simulink model "pipeline_test25"  (Simulink 8.9)
settings: Solver=VariableStepAuto  StartTime=0.0  StopTime=190  RelTol=1e-3
libraries: xbsIndex_r4 x105
settings Model: Creator=jeenx  LastModifiedBy=jeenx
settings DataIOCC: LimitDataPoints=off  SaveFormat=Dataset  SignalLoggingSaveFormat=Dataset  ReturnWorkspaceOutputs=on
settings OptimizationCC: LifeSpan=auto
settings DebuggingCC: UnderspecifiedInitializationDetection=Simplified  MergeDetectMultiDrivingBlocksExec=error  FcnCallInpInsideContextMsg=error  StateNameClashWarn=none  SFUnexpectedBacktrackingDiag=error  SFNoUnconditionalDefaultTransitionDiag=error  SFExecutionAtInitializationDiag=warning
settings HardwareCC: ProdBitPerPointer=64  ProdBitPerSizeT=64  ProdBitPerPtrDiffT=64  ProdLargestAtomicFloat=Float  ProdIntDivRoundTo=Zero  ProdEndianess=LittleEndian  ProdWordSize=64  ProdHWDeviceType=Intel->x86-64 (Windows64)
settings ModelReferenceCC: PropagateSignalLabelsOutOfModel=on
settings SFSimCC: SimUseLocalCustomCode=on
settings RTWCC: RTWUseLocalCustomCode=on
settings GRTTargetCC: TargetLangStandard=C99 (ISO)  GeneratePreprocessorConditionals=Use local settings  CombineOutputUpdateFcns=on  GRTInterface=off
settings ConfigComp: CovMetricSettings=dwe  CovHtmlReporting=off  CovSaveCumulativeToWorkspaceVar=off  CovSaveSingleToWorkspaceVar=off  CovExternalEMLEnable=on

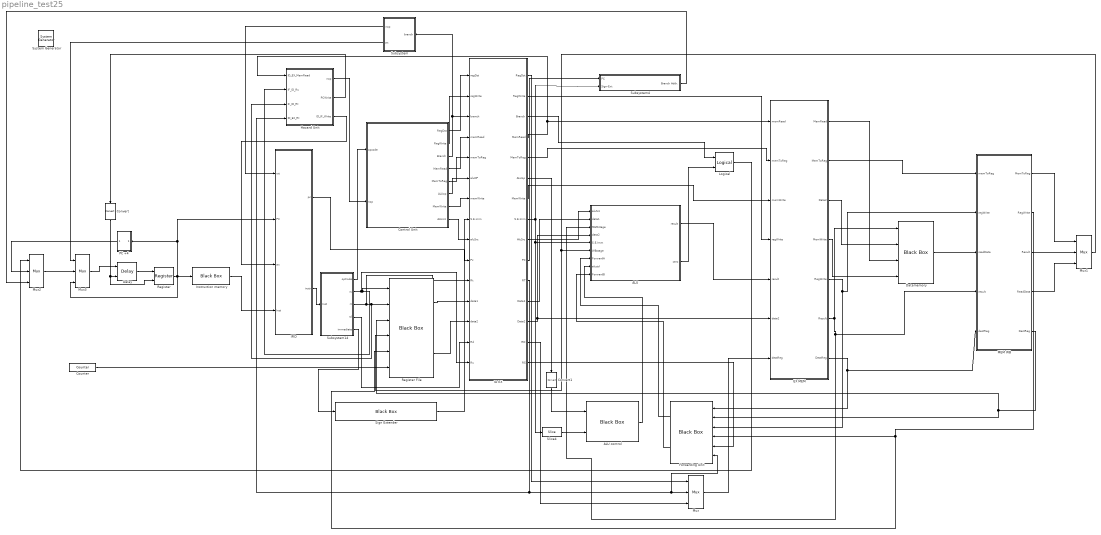
== system pipeline_test25 ==
  " System Generator" : xbsIndex_r4/ System Generator  Tag=genX  xilinxfamily=kintex7  part=xc7k325t  speed=-3  package=fbg676  synthesis_tool=Vivado  clock_wrapper=Clock Enables  directory=./netlist  proj_type=Vivado  Synth_file=Vivado Synthesis Defaults  Impl_file=Vivado Implementation Defaults  testbench=off  simulink_period=1  sysclk_period=10  dcm_input_clock_period=10  incr_netlist=off  trim_vbits=Everywhere in SubSystem  dbl_ovrd=According to Block Masks  core_generation=According to Block Masks  run_coregen=off  deprecated_control=off  eval_field=0  block_type=sysgen
  ALU : Subsystem
  ALU control : xbsIndex_r4/Black Box  init_code=ALU_control_config  sim_method=ISE Simulator  verbose=off  block_type=blackbox2
  Control Unit : Subsystem
  Convert : xbsIndex_r4/Convert  gui_display_data_type=Boolean  arith_type=Boolean  n_bits=16  bin_pt=14  float_type=Single  exp_bits=8  fraction_bits=24  quantization=Truncate  overflow=Wrap  en=off  latency=0  pipeline=off  dbl_ovrd=off  block_type=convert
  Convert1 : xbsIndex_r4/Convert  gui_display_data_type=Fixed-point  arith_type=Unsigned  n_bits=2  bin_pt=0  float_type=Single  exp_bits=8  fraction_bits=24  quantization=Truncate  overflow=Wrap  en=off  latency=0  pipeline=off  dbl_ovrd=off  block_type=convert
  Counter : xbsIndex_r4/Counter  cnt_type=Free Running  cnt_to=Inf  operation=Up  start_count=0  cnt_by_val=1  arith_type=Unsigned  n_bits=1  bin_pt=0  load_pin=off  rst=off  en=off  explicit_period=on  period=1  use_behavioral_HDL=off  implementation=Fabric  dbl_ovrd=off  block_type=counter
  Datamemory : xbsIndex_r4/Black Box  init_code=datamemory1_config  sim_method=ISE Simulator  verbose=off  block_type=blackbox2
  Delay : xbsIndex_r4/Delay  rst=off  infoeditControl=Selection of Reset will increase slice count due to use of real FFs and instead of SRLs  en=on  latency=1  reg_retiming=off  dbl_ovrd=off  block_type=delay
  EX MEM : Subsystem
  Forwarding Unit : xbsIndex_r4/Black Box  init_code=fw_u_config  sim_method=ISE Simulator  verbose=off  block_type=blackbox2
  Hazard Unit : Subsystem
  ID EX : Subsystem
  IFID : Subsystem
  Instruction memory : xbsIndex_r4/Black Box  init_code=instructionmemory_config  sim_method=ISE Simulator  verbose=off  block_type=blackbox2
  Logical : xbsIndex_r4/Logical  logical_function=AND  inputs=2  en=off  latency=0  precision=Full  arith_type=Unsigned  n_bits=16  bin_pt=0  align_bp=on  dbl_ovrd=off  block_type=logical
  MEM WB : Subsystem
  Mux : xbsIndex_r4/Mux  inputs=2  en=off  latency=0  precision=Full  arith_type=Unsigned  n_bits=16  bin_pt=14  quantization=Truncate  overflow=Wrap  dbl_ovrd=off  block_type=mux
  Mux1 : xbsIndex_r4/Mux  inputs=2  en=off  latency=0  precision=Full  arith_type=Unsigned  n_bits=16  bin_pt=14  quantization=Truncate  overflow=Wrap  dbl_ovrd=off  block_type=mux
  Mux2 : xbsIndex_r4/Mux  inputs=2  en=off  latency=0  precision=Full  arith_type=Unsigned  n_bits=32  bin_pt=0  quantization=Truncate  overflow=Wrap  dbl_ovrd=off  block_type=mux
  Mux3 : xbsIndex_r4/Mux  inputs=2  en=off  latency=0  precision=Full  arith_type=Unsigned  n_bits=16  bin_pt=14  quantization=Truncate  overflow=Wrap  dbl_ovrd=off  block_type=mux
  PC +4 : Subsystem
  Register : xbsIndex_r4/Register  init=0  rst=off  en=on  dbl_ovrd=off  block_type=register
  Register File : xbsIndex_r4/Black Box  init_code=regfile_config  sim_method=ISE Simulator  verbose=off  block_type=blackbox2
  Sign Extender : xbsIndex_r4/Black Box  init_code=SignExtender_config  sim_method=ISE Simulator  verbose=off  block_type=blackbox2
  Slice4 : xbsIndex_r4/Slice  nbits=6  boolean_output=off  mode=Lower Bit Location + Width  bit1=5  base1=Binary Point of Input  bit0=0  base0=LSB of Input  dbl_ovrd=off  block_type=slice
  Subsystem : Subsystem
  Subsystem14 : Subsystem
  Subsystem4 : Subsystem
  wires:
  EX MEM/1(MemRead) -> Datamemory/3
  ALU/1(result) -> EX MEM/5(result)
  MEM WB/2(RegWrite) -> Register File/5, Forwarding Unit/4
  Control Unit/3(Branch) -> ID EX/3(branch), Subsystem/1(branch)
  Sign Extender/1 -> ID EX/8(S.E.imm)
  Control Unit/5(MemToReg) -> ID EX/5(memToReg)
  EX MEM/4(MemWrite) -> Datamemory/4
  EX MEM/3(Data2) -> Datamemory/2
  Subsystem14/5(immediate) -> Sign Extender/1
  ID EX/15(RS) -> Forwarding Unit/5
  EX MEM/7(DestReg) -> Forwarding Unit/1, MEM WB/5(destReg)
  Slice4/1 -> ALU control/2
  Control Unit/2(RegWrite) -> ID EX/2(regWrite)
  Register File/1 -> ID EX/12(data1)
  Instruction memory/1 -> IFID/4(Inst)
  Convert1/1 -> ALU control/1
  ID EX/6(ALUop) -> Convert1/1
  ALU control/1 -> ALU/8(aluctrl)
  ALU/2(zero) -> Logical/2
  Convert/1 -> Register/2, Delay/2
  Control Unit/6(ALUop) -> ID EX/6(aluOP)
  ID EX/1(RegDst) -> Mux/1
  Hazard Unit/1(nop) -> Control Unit/2(nop)
  EX MEM/5(RegWrite) -> Forwarding Unit/3, MEM WB/2(regWrite)
  ID EX/7(MemWrite) -> EX MEM/3(memWrite)
  Subsystem/2(pc) -> Mux3/1
  ID EX/10(PC) -> Subsystem4/1(PC)
  Subsystem14/2(rs) -> ID EX/15(Rs), Hazard Unit/2(IF_ID_Rs), Register File/1
  Counter/1 -> Register File/6
  Forwarding Unit/1 -> ALU/7(ForwardA)
  Subsystem/1(nop) -> IFID/1(rst)
  Control Unit/4(MemRead) -> ID EX/4(memRead)
  MEM WB/5(DestReg) -> Register File/3, Forwarding Unit/2
  ID EX/11(RT) -> Hazard Unit/4(ID_EX_Rt), Forwarding Unit/6, Mux/2
  ID EX/3(Branch) -> Logical/1
  MEM WB/1(MemToReg) -> Mux1/1
  ID EX/4(MemRead) -> Hazard Unit/1(ID_EX_MemRead), EX MEM/1(memRead)
  Forwarding Unit/2 -> ALU/9(ForwardB)
  Datamemory/1 -> MEM WB/3(readData)
  ID EX/14(RD) -> Mux/3
  ID EX/12(Data1) -> ALU/2(data1)
  ID EX/5(MemToReg) -> EX MEM/2(memToReg)
  ID EX/13(Data2) -> EX MEM/6(data2), ALU/4(data2)
  EX MEM/2(MemToReg) -> MEM WB/1(memToReg)
  Mux3/1 -> Delay/1
  Subsystem14/1(opCode) -> Control Unit/1(opcode)
  Control Unit/1(RegDst) -> ID EX/1(regDst)
  Delay/1 -> Register/1
  ID EX/8(S.E.Imm) -> Subsystem4/2(Sign-Ext), Slice4/1, ALU/5(S.E.Imm)
  Mux1/1 -> Register File/4, ALU/6(WBstage)
  Mux2/1 -> Mux3/2
  Mux/1 -> EX MEM/7(destReg)
  Register/1 -> Instruction memory/1, Mux3/3, PC +4/1(In1), IFID/2(PC)
  MEM WB/3(Result) -> Mux1/2
  Subsystem14/3(rt) -> ID EX/11(Rt), Hazard Unit/3(IF_ID_Rt), Register File/2
  ID EX/2(RegWrite) -> EX MEM/4(regWrite)
  EX MEM/6(Result) -> MEM WB/4(result), ALU/3(MEMstage), Datamemory/1
  Hazard Unit/2(PCWrite) -> Convert/1
  IFID/2(instr) -> Subsystem14/1(Inst)
  Logical/1 -> Mux2/1
  Hazard Unit/3(ID_IF_Write) -> IFID/3(en)
  Subsystem14/4(rd) -> ID EX/14(Rd)
  Control Unit/8(ALUsrc) -> ID EX/9(aluSrc)
  Subsystem4/1(Branch Addr.) -> Mux2/3
  Register File/2 -> ID EX/13(data2)
  MEM WB/4(ReadData) -> Mux1/3
  ID EX/9(AluSrc) -> ALU/1(aluSrc)
  Control Unit/7(MemWrite) -> ID EX/7(memWrite)
  IFID/1(pc) -> ID EX/10(Pc)
  PC +4/1(Out1) -> Mux2/2

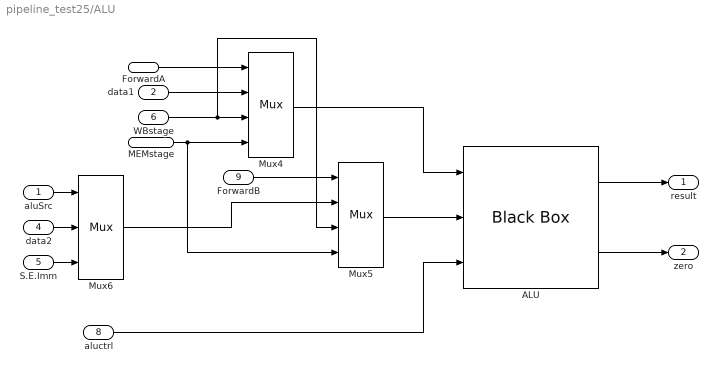
== system pipeline_test25/ALU ==
  aluSrc : Inport
  data1 : Inport  Port=2
  MEMstage : Inport  Port=3
  data2 : Inport  Port=4
  S.E.Imm : Inport  Port=5
  WBstage : Inport  Port=6
  ForwardA : Inport  Port=7
  aluctrl : Inport  Port=8
  ForwardB : Inport  Port=9
  ALU : xbsIndex_r4/Black Box  init_code=myalu_config  sim_method=ISE Simulator  verbose=off  block_type=blackbox2
  Mux4 : xbsIndex_r4/Mux  inputs=3  en=off  latency=0  precision=Full  arith_type=Unsigned  n_bits=16  bin_pt=14  quantization=Truncate  overflow=Wrap  dbl_ovrd=off  block_type=mux
  Mux5 : xbsIndex_r4/Mux  inputs=3  en=off  latency=0  precision=Full  arith_type=Unsigned  n_bits=16  bin_pt=14  quantization=Truncate  overflow=Wrap  dbl_ovrd=off  block_type=mux
  Mux6 : xbsIndex_r4/Mux  inputs=2  en=off  latency=0  precision=Full  arith_type=Unsigned  n_bits=16  bin_pt=14  quantization=Truncate  overflow=Wrap  dbl_ovrd=off  block_type=mux
  result : Outport
  zero : Outport  Port=2
  wires:
  ALU/1 -> result/1
  ALU/2 -> zero/1
  ForwardA/1 -> Mux4/1
  data1/1 -> Mux4/2
  MEMstage/1 -> Mux5/4, Mux4/4
  aluSrc/1 -> Mux6/1
  data2/1 -> Mux6/2
  S.E.Imm/1 -> Mux6/3
  aluctrl/1 -> ALU/3
  ForwardB/1 -> Mux5/1
  WBstage/1 -> Mux5/3, Mux4/3
  Mux6/1 -> Mux5/2
  Mux5/1 -> ALU/2
  Mux4/1 -> ALU/1

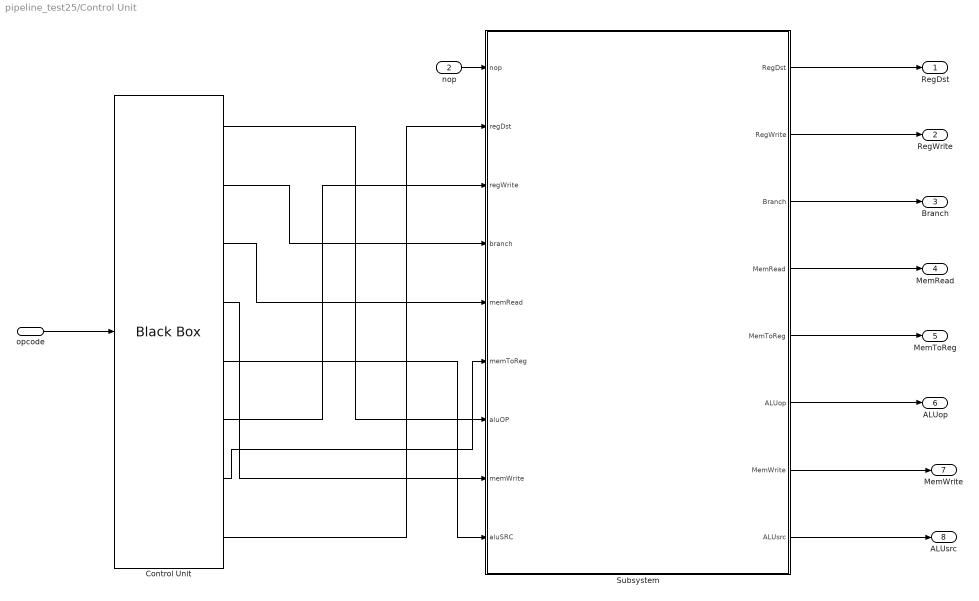
== system pipeline_test25/Control Unit ==
  opcode : Inport
  nop : Inport  Port=2
  Control Unit : xbsIndex_r4/Black Box  init_code=Control_unit_config  sim_method=ISE Simulator  verbose=off  block_type=blackbox2
  Subsystem : Subsystem
  RegDst : Outport
  RegWrite : Outport  Port=2
  Branch : Outport  Port=3
  MemRead : Outport  Port=4
  MemToReg : Outport  Port=5
  ALUop : Outport  Port=6
  MemWrite : Outport  Port=7
  ALUsrc : Outport  Port=8
  wires:
  Subsystem/5(MemToReg) -> MemToReg/1
  Subsystem/7(MemWrite) -> MemWrite/1
  Subsystem/2(RegWrite) -> RegWrite/1
  Subsystem/4(MemRead) -> MemRead/1
  Subsystem/6(ALUop) -> ALUop/1
  Subsystem/3(Branch) -> Branch/1
  Subsystem/1(RegDst) -> RegDst/1
  Subsystem/8(ALUsrc) -> ALUsrc/1
  opcode/1 -> Control Unit/1
  Control Unit/1 -> Subsystem/7(aluOP)
  Control Unit/2 -> Subsystem/4(branch)
  Control Unit/3 -> Subsystem/5(memRead)
  Control Unit/4 -> Subsystem/8(memWrite)
  Control Unit/5 -> Subsystem/9(aluSRC)
  Control Unit/6 -> Subsystem/3(regWrite)
  Control Unit/7 -> Subsystem/6(memToReg)
  Control Unit/8 -> Subsystem/2(regDst)
  nop/1 -> Subsystem/1(nop)

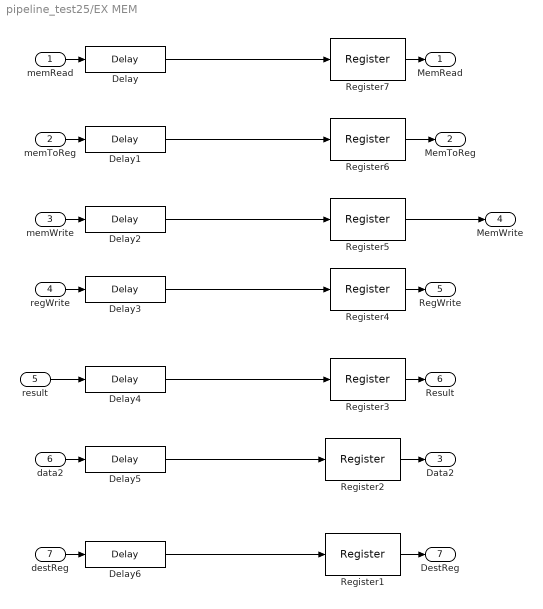
== system pipeline_test25/EX MEM ==
  memRead : Inport
  memToReg : Inport  Port=2
  memWrite : Inport  Port=3
  regWrite : Inport  Port=4
  result : Inport  Port=5
  data2 : Inport  Port=6
  destReg : Inport  Port=7
  Delay{,1..6} (7 alike) : xbsIndex_r4/Delay  rst=off  infoeditControl=Selection of Reset will increase slice count due to use of real FFs and instead of SRLs  en=off  latency=1  reg_retiming=off  dbl_ovrd=off  block_type=delay
  Register{1..7} (7 alike) : xbsIndex_r4/Register  init=0  rst=off  en=off  dbl_ovrd=off  block_type=register
  MemRead : Outport
  MemToReg : Outport  Port=2
  Data2 : Outport  Port=3
  MemWrite : Outport  Port=4
  RegWrite : Outport  Port=5
  Result : Outport  Port=6
  DestReg : Outport  Port=7
  wires:
  Delay1/1 -> Register6/1
  Delay/1 -> Register7/1
  memToReg/1 -> Delay1/1
  result/1 -> Delay4/1
  Register6/1 -> MemToReg/1
  regWrite/1 -> Delay3/1
  memRead/1 -> Delay/1
  destReg/1 -> Delay6/1
  data2/1 -> Delay5/1
  memWrite/1 -> Delay2/1
  Register7/1 -> MemRead/1
  Delay6/1 -> Register1/1
  Delay3/1 -> Register4/1
  Delay4/1 -> Register3/1
  Delay2/1 -> Register5/1
  Delay5/1 -> Register2/1
  Register5/1 -> MemWrite/1
  Register4/1 -> RegWrite/1
  Register3/1 -> Result/1
  Register2/1 -> Data2/1
  Register1/1 -> DestReg/1

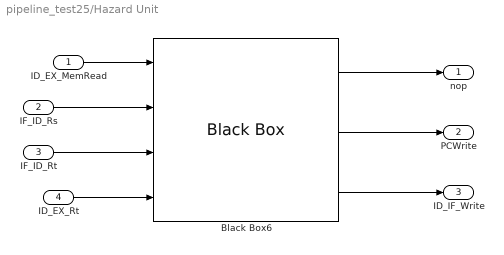
== system pipeline_test25/Hazard Unit ==
  ID_EX_MemRead : Inport
  IF_ID_Rs : Inport  Port=2
  IF_ID_Rt : Inport  Port=3
  ID_EX_Rt : Inport  Port=4
  Black Box6 : xbsIndex_r4/Black Box  init_code=Hazard_unit_config  sim_method=ISE Simulator  verbose=off  block_type=blackbox2
  nop : Outport
  PCWrite : Outport  Port=2
  ID_IF_Write : Outport  Port=3
  wires:
  Black Box6/3 -> ID_IF_Write/1
  ID_EX_MemRead/1 -> Black Box6/1
  IF_ID_Rs/1 -> Black Box6/2
  IF_ID_Rt/1 -> Black Box6/3
  ID_EX_Rt/1 -> Black Box6/4
  Black Box6/1 -> nop/1
  Black Box6/2 -> PCWrite/1

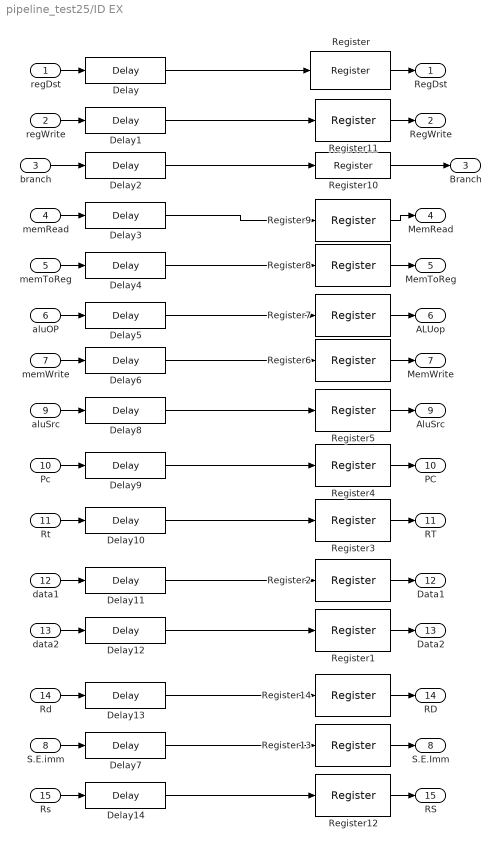
== system pipeline_test25/ID EX ==
  regDst : Inport
  regWrite : Inport  Port=2
  branch : Inport  Port=3
  memRead : Inport  Port=4
  memToReg : Inport  Port=5
  aluOP : Inport  Port=6
  memWrite : Inport  Port=7
  S.E.imm : Inport  Port=8
  aluSrc : Inport  Port=9
  Pc : Inport  Port=10
  Rt : Inport  Port=11
  data1 : Inport  Port=12
  data2 : Inport  Port=13
  Rd : Inport  Port=14
  Rs : Inport  Port=15
  Delay{,1..14} (15 alike) : xbsIndex_r4/Delay  rst=off  infoeditControl=Selection of Reset will increase slice count due to use of real FFs and instead of SRLs  en=off  latency=1  reg_retiming=off  dbl_ovrd=off  block_type=delay
  Register{,1..14} (15 alike) : xbsIndex_r4/Register  init=0  rst=off  en=off  dbl_ovrd=off  block_type=register
  RegDst : Outport
  RegWrite : Outport  Port=2
  Branch : Outport  Port=3
  MemRead : Outport  Port=4
  MemToReg : Outport  Port=5
  ALUop : Outport  Port=6
  MemWrite : Outport  Port=7
  S.E.Imm : Outport  Port=8
  AluSrc : Outport  Port=9
  PC : Outport  Port=10
  RT : Outport  Port=11
  Data1 : Outport  Port=12
  Data2 : Outport  Port=13
  RD : Outport  Port=14
  RS : Outport  Port=15
  wires:
  Delay2/1 -> Register10/1
  Delay6/1 -> Register6/1
  regWrite/1 -> Delay1/1
  Delay13/1 -> Register14/1
  Rt/1 -> Delay10/1
  memToReg/1 -> Delay4/1
  Delay12/1 -> Register1/1
  regDst/1 -> Delay/1
  branch/1 -> Delay2/1
  Rs/1 -> Delay14/1
  data1/1 -> Delay11/1
  memWrite/1 -> Delay6/1
  aluSrc/1 -> Delay8/1
  aluOP/1 -> Delay5/1
  Rd/1 -> Delay13/1
  memRead/1 -> Delay3/1
  data2/1 -> Delay12/1
  Register14/1 -> RD/1
  Pc/1 -> Delay9/1
  Register12/1 -> RS/1
  S.E.imm/1 -> Delay7/1
  Register8/1 -> MemToReg/1
  Register6/1 -> MemWrite/1
  Register10/1 -> Branch/1
  Register9/1 -> MemRead/1
  Register4/1 -> PC/1
  Register11/1 -> RegWrite/1
  Register7/1 -> ALUop/1
  Register13/1 -> S.E.Imm/1
  Register5/1 -> AluSrc/1
  Register/1 -> RegDst/1
  Register1/1 -> Data2/1
  Register2/1 -> Data1/1
  Register3/1 -> RT/1
  Delay4/1 -> Register8/1
  Delay11/1 -> Register2/1
  Delay3/1 -> Register9/1
  Delay8/1 -> Register5/1
  Delay7/1 -> Register13/1
  Delay14/1 -> Register12/1
  Delay5/1 -> Register7/1
  Delay/1 -> Register/1
  Delay9/1 -> Register4/1
  Delay1/1 -> Register11/1
  Delay10/1 -> Register3/1

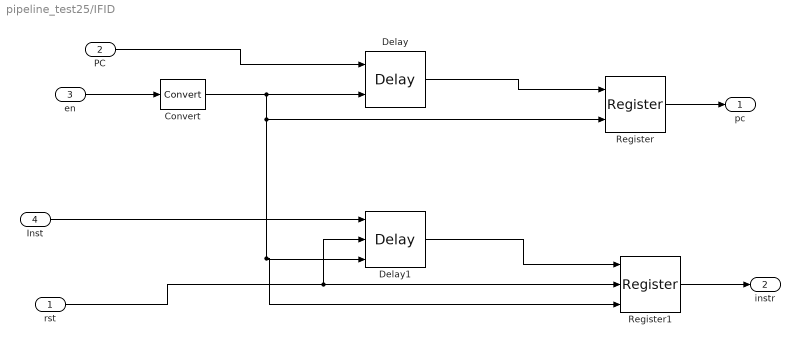
== system pipeline_test25/IFID ==
  rst : Inport
  PC : Inport  Port=2
  en : Inport  Port=3
  Inst : Inport  Port=4
  Convert : xbsIndex_r4/Convert  gui_display_data_type=Boolean  arith_type=Boolean  n_bits=1  bin_pt=0  float_type=Single  exp_bits=8  fraction_bits=24  quantization=Truncate  overflow=Wrap  en=off  latency=0  pipeline=off  dbl_ovrd=off  block_type=convert
  Delay : xbsIndex_r4/Delay  rst=off  infoeditControl=Selection of Reset will increase slice count due to use of real FFs and instead of SRLs  en=on  latency=1  reg_retiming=off  dbl_ovrd=off  block_type=delay
  Delay1 : xbsIndex_r4/Delay  rst=on  infoeditControl=Selection of Reset will increase slice count due to use of real FFs and instead of SRLs  en=on  latency=1  reg_retiming=off  dbl_ovrd=off  block_type=delay
  Register : xbsIndex_r4/Register  init=0  rst=off  en=on  dbl_ovrd=off  block_type=register
  Register1 : xbsIndex_r4/Register  init=0  rst=on  en=on  dbl_ovrd=off  block_type=register
  pc : Outport
  instr : Outport  Port=2
  wires:
  en/1 -> Convert/1
  Delay/1 -> Register/1
  rst/1 -> Delay1/2, Register1/2
  PC/1 -> Delay/1
  Inst/1 -> Delay1/1
  Register1/1 -> instr/1
  Register/1 -> pc/1
  Delay1/1 -> Register1/1
  Convert/1 -> Register1/3, Delay1/3, Register/2, Delay/2

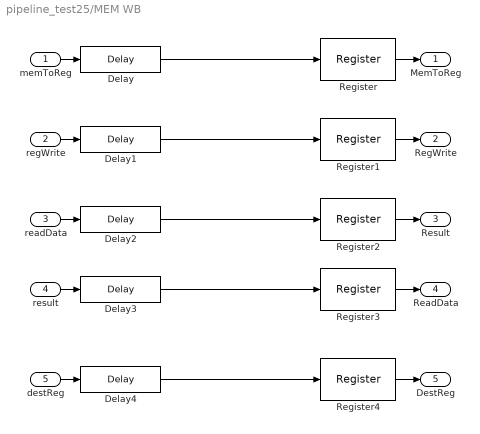
== system pipeline_test25/MEM WB ==
  memToReg : Inport
  regWrite : Inport  Port=2
  readData : Inport  Port=3
  result : Inport  Port=4
  destReg : Inport  Port=5
  Delay{,1..4} (5 alike) : xbsIndex_r4/Delay  rst=off  infoeditControl=Selection of Reset will increase slice count due to use of real FFs and instead of SRLs  en=off  latency=1  reg_retiming=off  dbl_ovrd=off  block_type=delay
  Register{,1..4} (5 alike) : xbsIndex_r4/Register  init=0  rst=off  en=off  dbl_ovrd=off  block_type=register
  MemToReg : Outport
  RegWrite : Outport  Port=2
  Result : Outport  Port=3
  ReadData : Outport  Port=4
  DestReg : Outport  Port=5
  wires:
  Delay/1 -> Register/1
  Delay1/1 -> Register1/1
  Delay2/1 -> Register2/1
  Delay4/1 -> Register4/1
  Delay3/1 -> Register3/1
  Register/1 -> MemToReg/1
  result/1 -> Delay3/1
  Register1/1 -> RegWrite/1
  Register2/1 -> Result/1
  destReg/1 -> Delay4/1
  Register4/1 -> DestReg/1
  readData/1 -> Delay2/1
  memToReg/1 -> Delay/1
  Register3/1 -> ReadData/1
  regWrite/1 -> Delay1/1

== system pipeline_test25/PC +4 ==
  In1 : Inport
  AddSub : xbsIndex_r4/AddSub  mode=Addition  use_carryin=off  use_carryout=off  en=off  latency=0  precision=User Defined  arith_type=Unsigned  n_bits=32  bin_pt=0  quantization=Truncate  overflow=Wrap  use_behavioral_HDL=off  hw_selection=Fabric  pipelined=off  dbl_ovrd=off  block_type=addsub
  Constant : xbsIndex_r4/Constant  const=4  gui_display_data_type=Fixed-point  arith_type=Unsigned  n_bits=32  bin_pt=0  preci_type=Single  exp_width=8  frac_width=24  explicit_period=on  period=1  equ=P=C  opselect=C  inp2=PCIN>>17  opr=+  inp1=P  carry=CIN  dbl_ovrd=off  block_type=constant
  Out1 : Outport
  wires:
  In1/1 -> AddSub/1
  Constant/1 -> AddSub/2
  AddSub/1 -> Out1/1

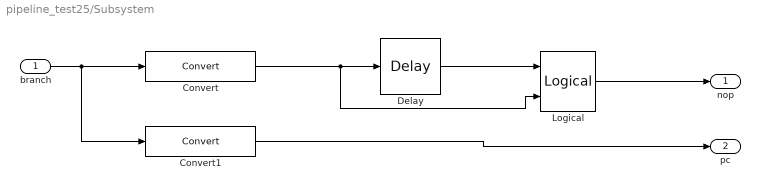
== system pipeline_test25/Subsystem ==
  branch : Inport
  Convert : xbsIndex_r4/Convert  gui_display_data_type=Boolean  arith_type=Boolean  n_bits=4  bin_pt=0  float_type=Single  exp_bits=8  fraction_bits=24  quantization=Truncate  overflow=Wrap  en=off  latency=0  pipeline=off  dbl_ovrd=off  block_type=convert
  Convert1 : xbsIndex_r4/Convert  gui_display_data_type=Boolean  arith_type=Boolean  n_bits=4  bin_pt=0  float_type=Single  exp_bits=8  fraction_bits=24  quantization=Truncate  overflow=Wrap  en=off  latency=0  pipeline=off  dbl_ovrd=off  block_type=convert
  Delay : xbsIndex_r4/Delay  rst=off  infoeditControl=Selection of Reset will increase slice count due to use of real FFs and instead of SRLs  en=off  latency=1  reg_retiming=off  dbl_ovrd=off  block_type=delay
  Logical : xbsIndex_r4/Logical  logical_function=OR  inputs=2  en=off  latency=1  precision=Full  arith_type=Unsigned  n_bits=16  bin_pt=0  align_bp=on  dbl_ovrd=off  block_type=logical
  nop : Outport
  pc : Outport  Port=2
  wires:
  Delay/1 -> Logical/1
  Logical/1 -> nop/1
  Convert1/1 -> pc/1
  Convert/1 -> Logical/2, Delay/1
  branch/1 -> Convert1/1, Convert/1

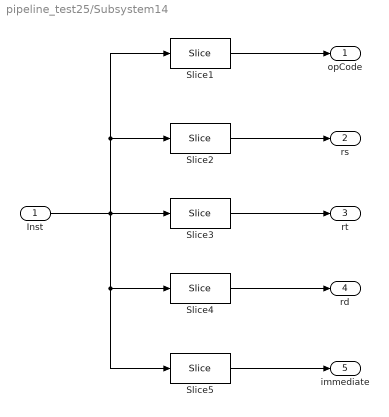
== system pipeline_test25/Subsystem14 ==
  Inst : Inport
  Slice1 : xbsIndex_r4/Slice  nbits=6  boolean_output=off  mode=Lower Bit Location + Width  bit1=0  base1=MSB of Input  bit0=26  base0=LSB of Input  dbl_ovrd=off  block_type=slice
  Slice2 : xbsIndex_r4/Slice  nbits=5  boolean_output=off  mode=Lower Bit Location + Width  bit1=0  base1=MSB of Input  bit0=21  base0=LSB of Input  dbl_ovrd=off  block_type=slice
  Slice3 : xbsIndex_r4/Slice  nbits=5  boolean_output=off  mode=Lower Bit Location + Width  bit1=0  base1=MSB of Input  bit0=16  base0=LSB of Input  dbl_ovrd=off  block_type=slice
  Slice4 : xbsIndex_r4/Slice  nbits=5  boolean_output=off  mode=Lower Bit Location + Width  bit1=0  base1=MSB of Input  bit0=11  base0=LSB of Input  dbl_ovrd=off  block_type=slice
  Slice5 : xbsIndex_r4/Slice  nbits=16  boolean_output=off  mode=Lower Bit Location + Width  bit1=0  base1=MSB of Input  bit0=0  base0=LSB of Input  dbl_ovrd=off  block_type=slice
  opCode : Outport
  rs : Outport  Port=2
  rt : Outport  Port=3
  rd : Outport  Port=4
  immediate : Outport  Port=5
  wires:
  Inst/1 -> Slice3/1, Slice4/1, Slice5/1, Slice2/1, Slice1/1
  Slice5/1 -> immediate/1
  Slice4/1 -> rd/1
  Slice3/1 -> rt/1
  Slice2/1 -> rs/1
  Slice1/1 -> opCode/1

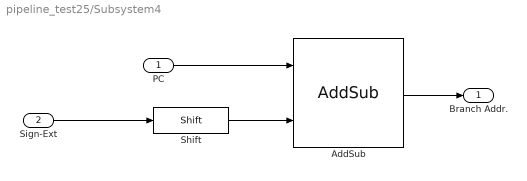
== system pipeline_test25/Subsystem4 ==
  PC : Inport
  Sign-Ext : Inport  Port=2
  AddSub : xbsIndex_r4/AddSub  mode=Addition  use_carryin=off  use_carryout=off  en=off  latency=0  precision=User Defined  arith_type=Unsigned  n_bits=32  bin_pt=0  quantization=Truncate  overflow=Wrap  use_behavioral_HDL=off  hw_selection=Fabric  pipelined=off  dbl_ovrd=off  block_type=addsub
  Shift : xbsIndex_r4/Shift  shift_dir=Left  shift_bits=2  en=off  latency=0  precision=Full  arith_type="Signed  (2's comp)"  n_bits=16  bin_pt=14  quantization=Truncate  overflow=Wrap  dbl_ovrd=off  block_type=shift
  Branch Addr. : Outport
  wires:
  Shift/1 -> AddSub/2
  Sign-Ext/1 -> Shift/1
  AddSub/1 -> Branch Addr./1
  PC/1 -> AddSub/1

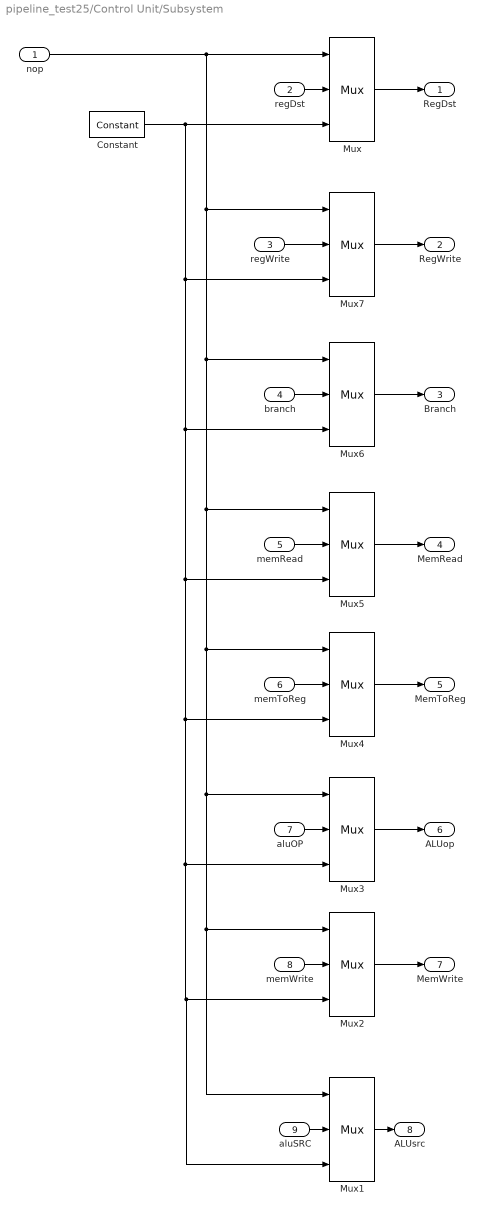
== system pipeline_test25/Control Unit/Subsystem ==
  nop : Inport
  regDst : Inport  Port=2
  regWrite : Inport  Port=3
  branch : Inport  Port=4
  memRead : Inport  Port=5
  memToReg : Inport  Port=6
  aluOP : Inport  Port=7
  memWrite : Inport  Port=8
  aluSRC : Inport  Port=9
  Constant : xbsIndex_r4/Constant  const=0  gui_display_data_type=Fixed-point  arith_type=Unsigned  n_bits=1  bin_pt=0  preci_type=Single  exp_width=8  frac_width=24  explicit_period=off  period=1  equ=P=C  opselect=C  inp2=PCIN>>17  opr=+  inp1=P  carry=CIN  dbl_ovrd=off  block_type=constant
  Mux{,1..7} (8 alike) : xbsIndex_r4/Mux  inputs=2  en=off  latency=0  precision=Full  arith_type=Unsigned  n_bits=16  bin_pt=14  quantization=Truncate  overflow=Wrap  dbl_ovrd=off  block_type=mux
  RegDst : Outport
  RegWrite : Outport  Port=2
  Branch : Outport  Port=3
  MemRead : Outport  Port=4
  MemToReg : Outport  Port=5
  ALUop : Outport  Port=6
  MemWrite : Outport  Port=7
  ALUsrc : Outport  Port=8
  wires:
  aluSRC/1 -> Mux1/2
  Mux1/1 -> ALUsrc/1
  Mux4/1 -> MemToReg/1
  Constant/1 -> Mux7/3, Mux6/3, Mux5/3, Mux4/3, Mux3/3, Mux1/3, Mux2/3, Mux/3
  Mux6/1 -> Branch/1
  regDst/1 -> Mux/2
  Mux5/1 -> MemRead/1
  memWrite/1 -> Mux2/2
  memToReg/1 -> Mux4/2
  Mux2/1 -> MemWrite/1
  Mux7/1 -> RegWrite/1
  aluOP/1 -> Mux3/2
  branch/1 -> Mux6/2
  Mux/1 -> RegDst/1
  regWrite/1 -> Mux7/2
  memRead/1 -> Mux5/2
  nop/1 -> Mux7/1, Mux6/1, Mux5/1, Mux4/1, Mux3/1, Mux1/1, Mux2/1, Mux/1
  Mux3/1 -> ALUop/1
